simulink model "Maglev_NMPC_Simscape"  (R2025a)
settings: Solver=ode23t  StartTime=0.0  StopTime=T_sim  FixedStep=mpc.Ts  MaxStep=0.0001  RelTol=1e-4
PreLoadFcn:
  | modelPath = fileparts(which(bdroot));
  | projectRoot = fileparts(modelPath);
  | 
  | run(fullfile(projectRoot, 'setup_sim_params.m'));
  | load(fullfile(projectRoot, 'Controller_Params', 'StandardNMPCData.mat'));
  | % Add the generated code folder so Simulink can find the mexw64
  | addpath(fullfile(projectRoot, 'Controller_Design/design_nmpc/c_generated_code'))
  | addpath(fullfile(projectRoot, 'Controller_Design/design_nmpc/c_generated_code/singleMaglev_model'))
  | 
  | load('sfun_port_names')
undefined symbols (not defined in the file): airgap_soll, Ext_Fina_Val, Ext_Init_Val, grav, I_max, I_min, mass, nmpc, T_stp
libraries: fl_lib x11, nesl_utility x4
settings Model: Creator=Polarstern  LastModifiedBy=CelestialAurora

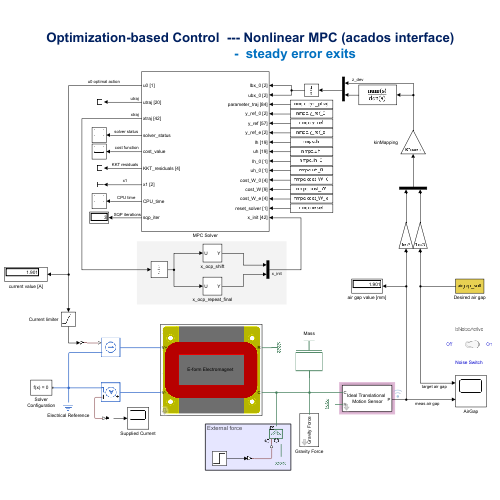
[thumbnail: Simulink's stored preview of the top-level diagram]
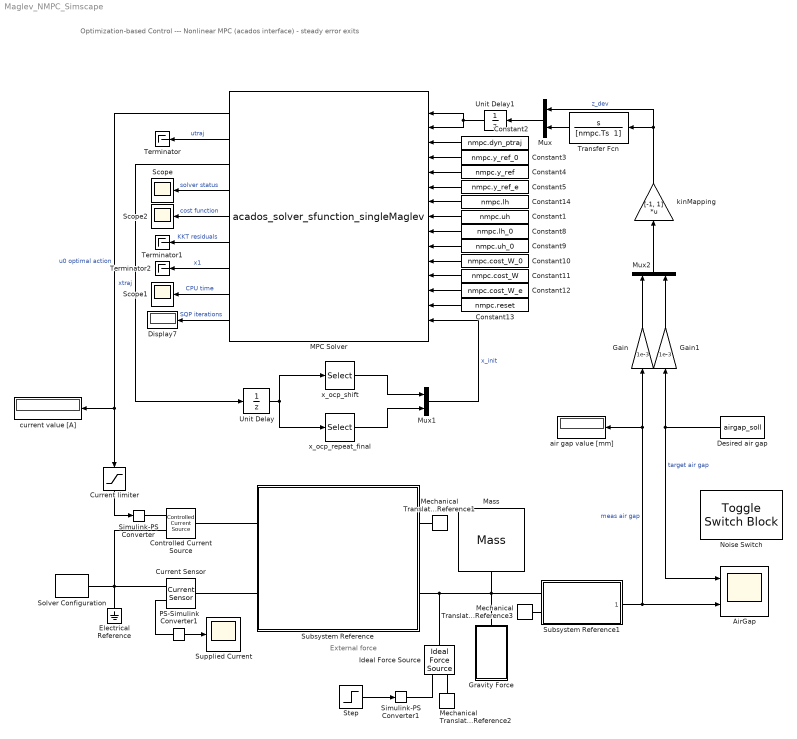
== system Maglev_NMPC_Simscape ==
  note: Optimization-based Control --- Nonlinear MPC (acados interface)
      | - steady error exits
  note: External force
  AirGap : Scope  NumInputPorts=2
      settings: ActiveDisplayYMinimum=1.7707247636659924  ActiveDisplayYMaximum=2.59428475461083
  Constant1 : Constant  Value=nmpc.uh
  Constant10 : Constant  Value=nmpc.cost_W_0
  Constant11 : Constant  Value=nmpc.cost_W
  Constant12 : Constant  Value=nmpc.cost_W_e
  Constant13 : Constant  Value=nmpc.reset
  Constant14 : Constant  Value=nmpc.lh
  Constant2 : Constant  Value=nmpc.dyn_ptraj
  Constant3 : Constant  Value=nmpc.y_ref_0
  Constant4 : Constant  Value=nmpc.y_ref
  Constant5 : Constant  Value=nmpc.y_ref_e
  Constant8 : Constant  Value=nmpc.lh_0
  Constant9 : Constant  Value=nmpc.uh_0
  Controlled Current Source : fl_lib/Electrical/Electrical Sources/Controlled Current Source
  Current Sensor : fl_lib/Electrical/Electrical Sensors/Current Sensor
  Current limiter : Saturate  UpperLimit=I_max  LowerLimit=I_min
  Desired air gap : Constant  Value=airgap_soll
  Display7 : Display
  Electrical Reference : fl_lib/Electrical/Electrical Elements/Electrical Reference
  Gain : Gain  Gain=1e-3
  Gain1 : Gain  Gain=1e-3
  Gravity Force : Subsystem
      mask DialogControl DescGroupVar Prompt: Gravity Force
      mask DialogControl DescTextVar Prompt: Fg = Mass*grav, as constant parameters predefined
      mask DialogControl DescTextVar2 Prompt: Direction: Downward
      mask Display: disp("Gravity Force")
  Ideal Force Source : fl_lib/Mechanical/Mechanical Sources/Ideal Force Source
  MPC Solver : S-Function  FunctionName=acados_solver_sfunction_singleMaglev  SFunctionDeploymentMode=off  EnableBusSupport=off
      mask Display:
      | global sfun_input_names sfun_output_names
      | for i = 1:length(sfun_input_names)
      | 	port_label('input', i, sfun_input_names{i})
      | end
      | for i = 1:length(sfun_output_names)
      | 	port_label('output', i, sfun_output_names{i})
      | end
  Mass : fl_lib/Mechanical/Translational Elements/Mass  mass=mass kg  num_ports=foundation.enum.numPorts2.one  v_specify=on  v_priority=Low  v=0 m/s  v_nominal_specify=off  v_nominal_value=1  v_nominal_unit=m/s  f_specify=off  f_priority=None  f=0 N  f_nominal_specify=off  f_nominal_value=700  f_nominal_unit=N
  Mechanical Translational Reference1 : fl_lib/Mechanical/Translational Elements/Mechanical Translational Reference
  Mechanical Translational Reference2 : fl_lib/Mechanical/Translational Elements/Mechanical Translational Reference
  Mechanical Translational Reference3 : fl_lib/Mechanical/Translational Elements/Mechanical Translational Reference
  Mux : Mux  Inputs=2
  Mux1 : Mux  Inputs=2
  Mux2 : Mux  Inputs=2
  Noise Switch : ToggleSwitchBlock
  PS-Simulink Converter1 : nesl_utility/PS-Simulink Converter  PhysicalDomain=network_engine_domain  SubClassName=ps_output  LeftPortType=input  RightPortType=output  PseudoPeriodic=off  Frequencies=[]  VectorFormat=inherit  Unit=inherit  AffineConversion=off
  Scope : Scope
      settings: ActiveDisplayYMinimum=-1  ActiveDisplayYMaximum=1
  Scope1 : Scope
      settings: ActiveDisplayYMinimum=-0.00038942499999999988  ActiveDisplayYMaximum=0.0041428249999999993  DataLoggingVariableName=ScopeData2
  Scope2 : Scope
      settings: ActiveDisplayYMinimum=-1  ActiveDisplayYMaximum=1  DataLoggingVariableName=ScopeData4
  Simulink-PS Converter : nesl_utility/Simulink-PS Converter  PhysicalDomain=network_engine_domain  SubClassName=ps_input  LeftPortType=input  RightPortType=output  PseudoPeriodic=off  Frequencies=[]  NoiseDistribution=none  NoiseParameters=[]  Unit=1  AffineConversion=off  FilteringAndDerivatives=zero  SimscapeFilterOrder=1  InputFilterTimeConstant=0.001  UdotUserProvided=0
  Simulink-PS Converter1 : nesl_utility/Simulink-PS Converter  PhysicalDomain=network_engine_domain  SubClassName=ps_input  LeftPortType=input  RightPortType=output  PseudoPeriodic=off  Frequencies=[]  NoiseDistribution=none  NoiseParameters=[]  Unit=1  AffineConversion=off  FilteringAndDerivatives=provide  SimscapeFilterOrder=1  InputFilterTimeConstant=0.001  UdotUserProvided=0
  Solver Configuration : nesl_utility/Solver Configuration  PhysicalDomain=network_engine_domain  SubClassName=solver  LeftPortType=input  RightPortType=generic  Tones=[]  Harmonics=[]  SimulateNoise=off  Profile=off  UseLocalSampling=off  EnableSwitchedLinearOptims=on  FrequencyDomain=off  UseCCode=off  RelTol=0.001  AbsTol=1e-06  MinStep=1e-09  ToWorkspace=off  RevertToSquareIcSolve=off  NumHomotopyIterations=100  PhasorMode=off  PhasorModeNumHarmonics=1  ConsistencySolver=NEWTON_XTOL_AFTER_FTOL  IndexReductionMethod=DerivativeReplacement  DoDC=off  ResidualTolerance=1e-09  ConsistencyTolSource=GLOBAL  ConsistencyAbsTol=0.001  ConsistencyRelTol=0.001  ConsistencyTolFactor=0.001  UseLocalSolver=off  LocalSolverChoice=NE_BACKWARD_EULER_ADVANCER  ResolveIndetEquations=on  FunctionEvalNumThread=1  LocalSolverSampleTime=0.001  DoFixedCost=off  MaxNonlinIter=3  MaxModeIter=2  ComputeImpulses=off  ImpulseIterations=2  LinearAlgebra=auto  LinearAlgebraNumThread=0  EquationFormulation=NE_TIME_EF  DelaysMemoryBudget=1024  AutomaticFiltering=on  FilteringTimeConstant=0.001  PartitionStorageMethod=AS_NEEDED  PartitionMemoryBudget=1024  PartitionMethod=ROBUST  MultibodyUseLocalSolver=off  MultibodyLocalSolverChoice=ODE1  MultibodyLocalSolverSampleTime=0.001
  Step : Step  Time=T_stp  Before=Ext_Init_Val  After=Ext_Fina_Val  SampleTime=0
  Subsystem Reference : Subsystem  ReferencedSubsystem=IntegratedElectromagnet  l_airgap=airgap_init
  Subsystem Reference1 : Subsystem  ReferencedSubsystem=IdealTrans_MotionSensor  ns_sw=isNoiseActive  ns_pw=NoisePower  ts=Ts  init_pos=airgap_init
  Supplied Current : Scope
      settings: ActiveDisplayYMinimum=1.8518069961964392  ActiveDisplayYMaximum=3.0825216237750865  DataLoggingVariableName=ScopeData3
  Terminator : Terminator
  Terminator1 : Terminator
  Terminator2 : Terminator
  Transfer Fcn : TransferFcn  Numerator=[1 0]  Denominator="[nmpc.Ts  1]"
  Unit Delay : UnitDelay  InitialCondition=nmpc.x_init  SampleTime=nmpc.Ts  HasFrameUpgradeWarning=on
  Unit Delay1 : UnitDelay  InitialCondition=nmpc.x_init_con  SampleTime=0.0001  HasFrameUpgradeWarning=on
  air gap value [mm] : Display
      settings: Decimation=4
  current value [A] : Display
  kinMapping : Gain  Gain=[-1, 1]  Multiplication=Matrix(K*u) (u vector)
  x_ocp_repeat_final : Selector  IndexMode=Zero-based  InputPortWidth=(nmpc.N+1)*nmpc.nx  IndexOptions=Starting index (dialog)  Indices=nmpc.N*nmpc.nx  OutputSizes=nmpc.nx
  x_ocp_shift : Selector  IndexMode=Zero-based  InputPortWidth=(nmpc.N+1)*nmpc.nx  IndexOptions=Starting index (dialog)  Indices=nmpc.nx  OutputSizes=nmpc.N*nmpc.nx
  wires:
  MPC Solver/1 -> current value [A]/1, Current limiter/1  "u0 optimal action"
  MPC Solver/2 -> Terminator/1  "utraj"
  MPC Solver/3 -> Unit Delay/1  "xtraj"
  MPC Solver/4 -> Scope/1  "solver status"
  MPC Solver/5 -> Scope2/1  "cost function"
  MPC Solver/6 -> Terminator1/1  "KKT residuals"
  MPC Solver/7 -> Terminator2/1  "x1"
  MPC Solver/8 -> Scope1/1  "CPU time"
  MPC Solver/9 -> Display7/1  "SQP iterations"
  Unit Delay/1 -> x_ocp_repeat_final/1, x_ocp_shift/1
  x_ocp_repeat_final/1 -> Mux1/2
  x_ocp_shift/1 -> Mux1/1
  Constant2/1 -> MPC Solver/3
  Constant3/1 -> MPC Solver/4
  Constant4/1 -> MPC Solver/5
  Constant5/1 -> MPC Solver/6
  Constant14/1 -> MPC Solver/7
  Constant1/1 -> MPC Solver/8
  Constant8/1 -> MPC Solver/9
  Constant9/1 -> MPC Solver/10
  Constant10/1 -> MPC Solver/11
  Constant11/1 -> MPC Solver/12
  Constant12/1 -> MPC Solver/13
  Constant13/1 -> MPC Solver/14
  Mux1/1 -> MPC Solver/15  "x_init"
  Unit Delay1/1 -> MPC Solver/2, MPC Solver/1
  Mux2/1 -> kinMapping/1
  Desired air gap/1 -> AirGap/1, Gain1/1  "target air gap"
  Subsystem Reference1/1 -> AirGap/2, Gain/1, air gap value [mm]/1  "meas air gap"
  Step/1 -> Simulink-PS Converter1/1
  PS-Simulink Converter1/1 -> Supplied Current/1
  Current limiter/1 -> Simulink-PS Converter/1
  kinMapping/1 -> Mux/1, Transfer Fcn/1  "z_dev"
  Gain/1 -> Mux2/1
  Gain1/1 -> Mux2/2
  Mux/1 -> Unit Delay1/1
  Transfer Fcn/1 -> Mux/2
  connections:
  Controlled Current Source/RConn2 -- Solver Configuration/RConn1 -- Electrical Reference/LConn1 -- Current Sensor/RConn2
  Subsystem Reference/RConn2 -- Subsystem Reference1/LConn1 -- Gravity Force/RConn1 -- Mass/LConn1 -- Ideal Force Source/LConn1
  Mechanical Translational Reference3/LConn1 -- Subsystem Reference1/LConn2
  Subsystem Reference/LConn2 -- Current Sensor/LConn1
  Simulink-PS Converter1/RConn1 -- Ideal Force Source/RConn1
  Mechanical Translational Reference2/LConn1 -- Ideal Force Source/RConn2
  PS-Simulink Converter1/LConn1 -- Current Sensor/RConn1
  Subsystem Reference/RConn1 -- Mechanical Translational Reference1/LConn1
  Subsystem Reference/LConn1 -- Controlled Current Source/LConn1
  Simulink-PS Converter/RConn1 -- Controlled Current Source/RConn1

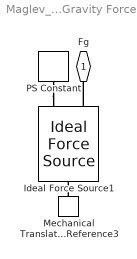
== system Maglev_NMPC_Simscape/Gravity Force ==
  Ideal Force Source1 : fl_lib/Mechanical/Mechanical Sources/Ideal Force Source
  Mechanical Translational Reference3 : fl_lib/Mechanical/Translational Elements/Mechanical Translational Reference
  PS Constant : fl_lib/Physical Signals/Sources/PS Constant  constant=mass*grav N
  Fg : PMIOPort  Side=Right
  connections:
  Mechanical Translational Reference3/LConn1 -- Ideal Force Source1/LConn1
  PS Constant/RConn1 -- Ideal Force Source1/RConn1
  Ideal Force Source1/RConn2 -- Fg/RConn1
